simulink model "PV_MEV"  (R2025a)
settings: Solver=VariableStepAuto  StartTime=0.0  StopTime=1  RelTol=1e-3
InitFcn:
  | init_paras
undefined symbols (not defined in the file): C_PFC, D1, Delta, DiscIntNeverNeededParam, ENABLE_HIL, estimation_src, Fnom, Fr_I, Ki_V, Kp_I, Kp_V, Kr_I, L_PFC, Limit_V, mm_10cycle_points, mm_fund_freq, mm_points_per_cycle, RL_PFC, Ro, Ts_Control, Ts_Power, use_d_predict, use_harmonic, use_p_predict, Vnom_ac
libraries: spsSeriesRLCBranchLib x17, spsMeanLib x16, spsCurrentMeasurementLib x9, spsFourierLib x8, spsTHDLib x8, spsVoltageMeasurementLib x8, spsDiodeLib x7, MyLibrary x6, instrumentlib x6, pycoexlib x6, simulink x6, spsPWMGeneratorDCDCLib x4
(part 3 of 6)

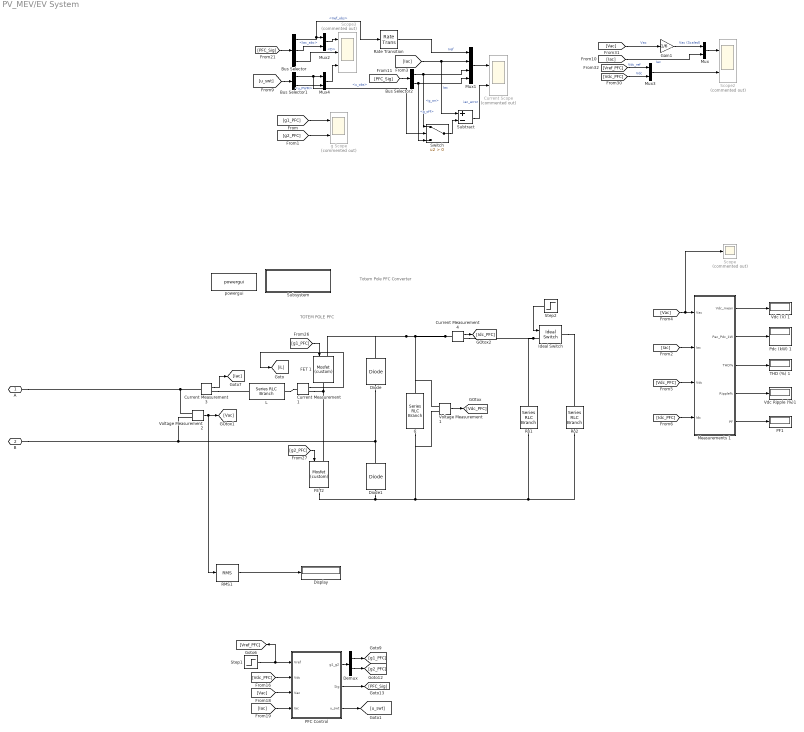
== system PV_MEV/EV System ==
  note: TOTEM POLE PFC
  note: Totem Pole PFC Converter
  Bus Selector : BusSelector  OutputSignals=Iref_obs,Iac_abc,D
  Bus Selector1 : BusSelector  OutputSignals=u_obs,u_PWM
  Bus Selector2 : BusSelector  OutputSignals=g_on,g_off
  C : spsSeriesRLCBranchLib/Series RLC Branch  LConnTagsString=__new0  RConnTagsString=__new0  BranchType=C  Resistance=1  Inductance=1e-3  SetiL0=off  InitialCurrent=0  Capacitance=C_PFC  Setx0=on  InitialVoltage=375  Measurements=None
  Current Measurement1 : spsCurrentMeasurementLib/Current Measurement  PhasorSimulation=off  OutputType=Complex  PSBequivalent=0
  Current Measurement3 : spsCurrentMeasurementLib/Current Measurement  PhasorSimulation=off  OutputType=Complex  PSBequivalent=0
  Current Measurement4 : spsCurrentMeasurementLib/Current Measurement  PhasorSimulation=off  OutputType=Complex  PSBequivalent=0
  Current Scope : Scope  Commented=on  NumInputPorts=2
      settings: ActiveDisplayYMinimum=-76.3871  ActiveDisplayYMaximum=79.5142  DataLoggingSaveFormat=Array
  Demux : Demux  Outputs=2
  Diode : spsDiodeLib/Diode  Ron=Ron_Diode  Lon=0  Vf=Vf  IC=0  UseSnubber=0  Rs=1e6  Cs=inf  Measurements=off
  Diode1 : spsDiodeLib/Diode  Ron=Ron_Diode  Lon=0  Vf=Vf  IC=0  UseSnubber=0  Rs=1e6  Cs=inf  Measurements=off
  Display : Display
  FET 1 : MyLibrary/Mosfet (custom)  Ron=Ron_FET  Lon=0  Rd=Ron_Diode  Vfd=Vf  IC=0  Rs=1e6  Cs=inf  Measurements=off
  FET2 : MyLibrary/Mosfet (custom)  Ron=Ron_FET  Lon=0  Rd=Ron_Diode  Vfd=Vf  IC=0  Rs=1e6  Cs=inf  Measurements=off
  Gain1 : Gain  Gain=1/6
  Ideal Switch : spsIdealSwitchLib/Ideal Switch  Ron=0.001  Lon=0  IC=0  Rs=1e5  Cs=inf  Measurements=off
  L : spsSeriesRLCBranchLib/Series RLC Branch  LConnTagsString=__new0  RConnTagsString=__new0  BranchType=RL  Resistance=RL_PFC  Inductance=L_PFC  SetiL0=off  InitialCurrent=0  Capacitance=1e-6  Setx0=off  InitialVoltage=0  Measurements=None
  Measurements 1 : Subsystem
  Mux{,2..4} (4 alike) : Mux  Inputs=2
  Mux1 : Mux
  PF1 : Display
      settings: Format=bank  Decimation=100
  PFC Control : Subsystem
  Pdc (kW) 1 : Display
      settings: Format=bank  Decimation=100
  RMS1 : spsRMSLib/RMS  TrueRMS=on  Freq=60  RMSInit=0  Ts=5E-08
  Rate Transition : RateTransition
  Ro1 : spsSeriesRLCBranchLib/Series RLC Branch  LConnTagsString=__new0  RConnTagsString=__new0  BranchType=R  Resistance=Ro*2  Inductance=200e-6  SetiL0=off  InitialCurrent=0  Capacitance=400e-6  Setx0=off  InitialVoltage=0  Measurements=None
  Ro2 : spsSeriesRLCBranchLib/Series RLC Branch  LConnTagsString=__new0  RConnTagsString=__new0  BranchType=R  Resistance=Ro*2  Inductance=200e-6  SetiL0=off  InitialCurrent=0  Capacitance=400e-6  Setx0=off  InitialVoltage=0  Measurements=None
  Scope : Scope  Commented=on
      settings: ActiveDisplayYMinimum=193.54878166788092  ActiveDisplayYMaximum=209.93761298828721  DataLoggingVariableName=ScopeData2  DataLoggingSaveFormat=Array
  Scope2 : Scope  Commented=on  NumInputPorts=2
      settings: ActiveDisplayYMinimum=-127.2219  ActiveDisplayYMaximum=127.2109  DataLoggingVariableName=ScopeData3  DataLoggingSaveFormat=Array
  Scope3 : Scope  Commented=on  NumInputPorts=3
      settings: ActiveDisplayYMinimum=-13.4274  ActiveDisplayYMaximum=110.8467  DataLoggingVariableName=ScopeData4  DataLoggingSaveFormat=Array
  Step1 : Step  Time=0.2  Before=350  After=400  SampleTime=Ts_Power
  Step2 : Step  Time=0.4  SampleTime=Ts_Power
  Subsystem : Subsystem
      settings: OpenFcn=edit('Totem_Pole_PFC_v1_data');
      mask Display: disp('Double-click to open\n parameters file');
  Subtract : Sum  Inputs=+-
  Switch : Switch  Criteria=u2 > Threshold  SaturateOnIntegerOverflow=off  InputSameDT=off
  THD (%) 1 : Display
      settings: Format=bank  Decimation=100
  Vdc (V) 1 : Display
      settings: Format=bank  Decimation=100
  Vdc Ripple (%)1 : Display
      settings: Format=bank  Decimation=100
  Voltage Measurement1 : spsVoltageMeasurementLib/Voltage Measurement  PhasorSimulation=off  OutputType=Complex  PSBequivalent=0
  Voltage Measurement2 : spsVoltageMeasurementLib/Voltage Measurement  PhasorSimulation=off  OutputType=Complex  PSBequivalent=0
  g Scope : Scope  Commented=on  NumInputPorts=2
      settings: ActiveDisplayYMinimum=-0.125  ActiveDisplayYMaximum=1.125  DataLoggingVariableName=ScopeData5  DataLoggingSaveFormat=Array
  powergui : spspowerguiLib/powergui  Priority=1  SimulationMode=Discrete  SampleTime=Ts_Power  frequency=60  Iterations=50  frequencyindice=0  Pbase=100e6  ErrMax=1e-4  UnitsV=kV  UnitsW=MW  buscounter=0  FunctionMessages=off  echomessages=off  EnableUseOfTLC=off  CurrentSourceSwitches=off  DisableSnubberDevices=off  DisableRonSwitches=off  DisableVfSwitches=off  DisplayEquations=off  AutomaticDiscreteSolvers=off  SolverType=Tustin/Backward Euler (TBE)  Interpol=off  ExternalGateDelay=off  methode=off  Ts=100  x0status=blocks  SPID=on  SwTol=0  HookPort=off  NonlinearTolerance=1e-4  nMaxIteration=100  ContinueOnMaxIteration=off  RestoreLinks=warning  ResistiveCurrentMeasurement=off  Frange=[0:2:500]  Ylog=off  Xlog=on  ShowGrid=off  save=off  variable=ZData  structure=0  ZoomFFT=off  StartTime=0.0  cycles=1  DisplayStyle=1  fundamental=60  FreqAxis=off  MaxFrequency=1000  frequencyindicesteady=1  RmsSteady=1  display=off
  A : PMIOPort  Side=Left
  B : PMIOPort  Port=2  Side=Left
  wires:
  Bus Selector1/1 -> Mux4/1, Switch/2  "<u_obs>"
  Bus Selector/2 -> Mux2/2  "<Iac_abc>"
  Step1/1 -> PFC Control/1(Vref), [Vref_PFC]
  [g2_PFC] -> FET2/1
  [Iac] -> Measurements 1/2(Iac)
  Bus Selector/3 -> Scope3/2  "<D>"
  [g1_PFC] -> g Scope/1
  Measurements 1/3(THD%) -> THD (%) 1/1
  Voltage Measurement2/1 -> RMS1/1, [Vac]
  Mux3/1 -> Scope2/2
  Measurements 1/4(Ripple%) -> Vdc Ripple (%)1/1
  PFC Control/1(g1_g2) -> Demux/1
  PFC Control/3(u_swt) -> [u_swt]
  Bus Selector2/2 -> Mux1/4, Switch/3  "<g_off>"
  Mux2/1 -> Scope3/1
  Measurements 1/2(Pac_Pdc_kW) -> Pdc (kW) 1/1
  Step2/1 -> Ideal Switch/1
  [Idc_PFC] -> Measurements 1/4(Idc)
  [Iac] -> Subtract/1, Mux1/2  "Iac"
  Gain1/1 -> Mux/1  "Vac (Scaled)"
  [u_swt] -> Bus Selector1/1
  Bus Selector/1 -> Rate Transition/1, Mux2/1  "<Iref_obs>"
  Measurements 1/1(Vdc_mean) -> Vdc (V) 1/1
  [g2_PFC] -> g Scope/2
  [PFC_Sig] -> Bus Selector2/1
  [Vac] -> Scope/1, Measurements 1/1(Vac)
  [Vac] -> Gain1/1  "Vac"
  PFC Control/2(Sig) -> [PFC_Sig]
  [PFC_Sig] -> Bus Selector/1
  [Vdc_PFC] -> PFC Control/2(Vdc)
  Voltage Measurement1/1 -> [Vdc_PFC]
  [g1_PFC] -> FET 1/1
  [Vac] -> PFC Control/3(Vac)
  [Vdc_PFC] -> Measurements 1/3(Vdc)
  Mux/1 -> Scope2/1
  Bus Selector1/2 -> Mux4/2  "<u_PWM>"
  RMS1/1 -> Display/1
  Current Measurement3/1 -> [Iac]
  [Iac] -> Mux/2  "Iac"
  Bus Selector2/1 -> Switch/1, Mux1/3  "<g_on>"
  Switch/1 -> Subtract/2
  Current Measurement1/1 -> [iL]
  [Iac] -> PFC Control/4(Iac)
  Mux4/1 -> Scope3/3
  [Vdc_PFC] -> Mux3/2  "Vdc"
  Demux/1 -> [g1_PFC]
  Demux/2 -> [g2_PFC]
  Rate Transition/1 -> Mux1/1  "Iref"
  Measurements 1/5(PF) -> PF1/1
  Mux1/1 -> Current Scope/1
  [Vref_PFC] -> Mux3/1  "Vdc_ref"
  Subtract/1 -> Current Scope/2  "iac_error"
  Current Measurement4/1 -> [Idc_PFC]
  connections:
  Ideal Switch/LConn1 -- Ro1/LConn1 -- Current Measurement4/RConn1
  Current Measurement1/RConn1 -- FET2/LConn1 -- FET 1/RConn1
  Ro2/RConn1 -- Ro1/RConn1 -- C/RConn1 -- Voltage Measurement1/LConn2 -- FET2/RConn1 -- Diode1/LConn1
  Voltage Measurement2/LConn2 -- B/RConn1 -- Diode/LConn1 -- Diode1/RConn1
  Current Measurement4/LConn1 -- Voltage Measurement1/LConn1 -- C/LConn1 -- Diode/RConn1 -- FET 1/LConn1
  Voltage Measurement2/LConn1 -- A/RConn1 -- Current Measurement3/LConn1
  Current Measurement3/RConn1 -- L/LConn1
  L/RConn1 -- Current Measurement1/LConn1
  Ideal Switch/RConn1 -- Ro2/LConn1

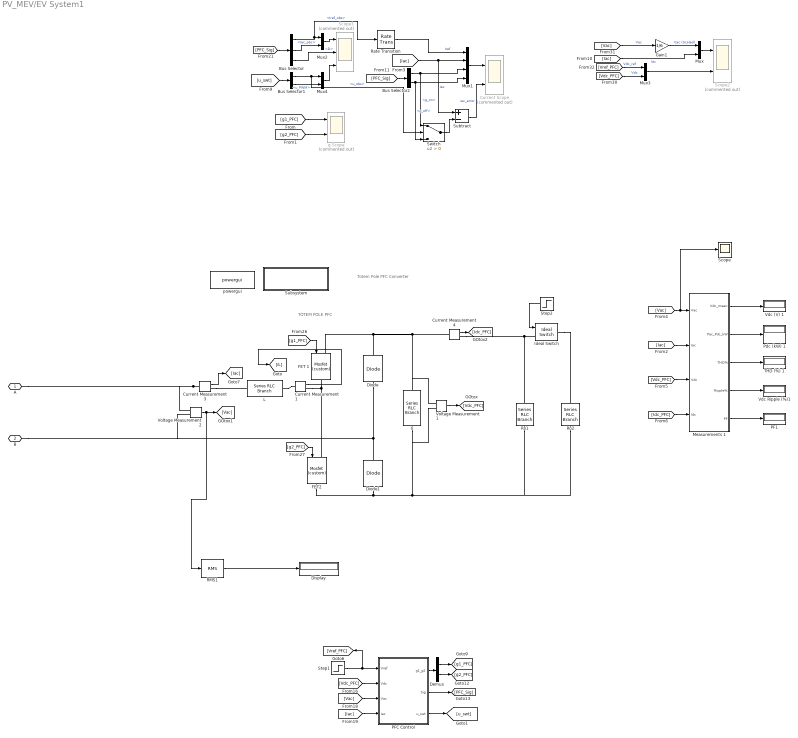
== system PV_MEV/EV System1 ==
  note: Totem Pole PFC Converter
  note: TOTEM POLE PFC
  Bus Selector : BusSelector  OutputSignals=Iref_obs,Iac_abc,D
  Bus Selector1 : BusSelector  OutputSignals=u_obs,u_PWM
  Bus Selector2 : BusSelector  OutputSignals=g_on,g_off
  C : spsSeriesRLCBranchLib/Series RLC Branch  LConnTagsString=__new0  RConnTagsString=__new0  BranchType=C  Resistance=1  Inductance=1e-3  SetiL0=off  InitialCurrent=0  Capacitance=C_PFC  Setx0=on  InitialVoltage=375  Measurements=None
  Current Measurement1 : spsCurrentMeasurementLib/Current Measurement  PhasorSimulation=off  OutputType=Complex  PSBequivalent=0
  Current Measurement3 : spsCurrentMeasurementLib/Current Measurement  PhasorSimulation=off  OutputType=Complex  PSBequivalent=0
  Current Measurement4 : spsCurrentMeasurementLib/Current Measurement  PhasorSimulation=off  OutputType=Complex  PSBequivalent=0
  Current Scope : Scope  Commented=on  NumInputPorts=2
      settings: ActiveDisplayYMinimum=-76.3871  ActiveDisplayYMaximum=79.5142  DataLoggingSaveFormat=Array
  Demux : Demux  Outputs=2
  Diode : spsDiodeLib/Diode  Ron=Ron_Diode  Lon=0  Vf=Vf  IC=0  UseSnubber=0  Rs=1e6  Cs=inf  Measurements=off
  Diode1 : spsDiodeLib/Diode  Ron=Ron_Diode  Lon=0  Vf=Vf  IC=0  UseSnubber=0  Rs=1e6  Cs=inf  Measurements=off
  Display : Display
  FET 1 : MyLibrary/Mosfet (custom)  Ron=Ron_FET  Lon=0  Rd=Ron_Diode  Vfd=Vf  IC=0  Rs=1e6  Cs=inf  Measurements=off
  FET2 : MyLibrary/Mosfet (custom)  Ron=Ron_FET  Lon=0  Rd=Ron_Diode  Vfd=Vf  IC=0  Rs=1e6  Cs=inf  Measurements=off
  Gain1 : Gain  Gain=1/6
  Ideal Switch : spsIdealSwitchLib/Ideal Switch  Ron=0.001  Lon=0  IC=0  Rs=1e5  Cs=inf  Measurements=off
  L : spsSeriesRLCBranchLib/Series RLC Branch  LConnTagsString=__new0  RConnTagsString=__new0  BranchType=RL  Resistance=RL_PFC  Inductance=L_PFC  SetiL0=off  InitialCurrent=0  Capacitance=1e-6  Setx0=off  InitialVoltage=0  Measurements=None
  Measurements 1 : Subsystem
  Mux{,2..4} (4 alike) : Mux  Inputs=2
  Mux1 : Mux
  PF1 : Display
      settings: Format=bank  Decimation=100
  PFC Control : Subsystem
  Pdc (kW) 1 : Display
      settings: Format=bank  Decimation=100
  RMS1 : spsRMSLib/RMS  TrueRMS=on  Freq=60  RMSInit=0  Ts=5E-08
  Rate Transition : RateTransition
  Ro1 : spsSeriesRLCBranchLib/Series RLC Branch  LConnTagsString=__new0  RConnTagsString=__new0  BranchType=R  Resistance=Ro*2  Inductance=200e-6  SetiL0=off  InitialCurrent=0  Capacitance=400e-6  Setx0=off  InitialVoltage=0  Measurements=None
  Ro2 : spsSeriesRLCBranchLib/Series RLC Branch  LConnTagsString=__new0  RConnTagsString=__new0  BranchType=R  Resistance=Ro*2  Inductance=200e-6  SetiL0=off  InitialCurrent=0  Capacitance=400e-6  Setx0=off  InitialVoltage=0  Measurements=None
  Scope : Scope
      settings: DataLoggingVariableName=ScopeData2  DataLoggingSaveFormat=Array
  Scope2 : Scope  Commented=on  NumInputPorts=2
      settings: ActiveDisplayYMinimum=-127.2219  ActiveDisplayYMaximum=127.2109  DataLoggingVariableName=ScopeData3  DataLoggingSaveFormat=Array
  Scope3 : Scope  Commented=on  NumInputPorts=3
      settings: ActiveDisplayYMinimum=-13.4274  ActiveDisplayYMaximum=110.8467  DataLoggingVariableName=ScopeData4  DataLoggingSaveFormat=Array
  Step1 : Step  Time=0.2  Before=350  After=400  SampleTime=Ts_Power
  Step2 : Step  Time=0.4  SampleTime=Ts_Power
  Subsystem : Subsystem
      settings: OpenFcn=edit('Totem_Pole_PFC_v1_data');
      mask Display: disp('Double-click to open\n parameters file');
  Subtract : Sum  Inputs=+-
  Switch : Switch  Criteria=u2 > Threshold  SaturateOnIntegerOverflow=off  InputSameDT=off
  THD (%) 1 : Display
      settings: Format=bank  Decimation=100
  Vdc (V) 1 : Display
      settings: Format=bank  Decimation=100
  Vdc Ripple (%)1 : Display
      settings: Format=bank  Decimation=100
  Voltage Measurement1 : spsVoltageMeasurementLib/Voltage Measurement  PhasorSimulation=off  OutputType=Complex  PSBequivalent=0
  Voltage Measurement2 : spsVoltageMeasurementLib/Voltage Measurement  PhasorSimulation=off  OutputType=Complex  PSBequivalent=0
  g Scope : Scope  Commented=on  NumInputPorts=2
      settings: ActiveDisplayYMinimum=-0.125  ActiveDisplayYMaximum=1.125  DataLoggingVariableName=ScopeData5  DataLoggingSaveFormat=Array
  powergui : spspowerguiLib/powergui  Priority=1  SimulationMode=Discrete  SampleTime=Ts_Power  frequency=60  Iterations=50  frequencyindice=0  Pbase=100e6  ErrMax=1e-4  UnitsV=kV  UnitsW=MW  buscounter=0  FunctionMessages=off  echomessages=off  EnableUseOfTLC=off  CurrentSourceSwitches=off  DisableSnubberDevices=off  DisableRonSwitches=off  DisableVfSwitches=off  DisplayEquations=off  AutomaticDiscreteSolvers=off  SolverType=Tustin/Backward Euler (TBE)  Interpol=off  ExternalGateDelay=off  methode=off  Ts=100  x0status=blocks  SPID=on  SwTol=0  HookPort=off  NonlinearTolerance=1e-4  nMaxIteration=100  ContinueOnMaxIteration=off  RestoreLinks=warning  ResistiveCurrentMeasurement=off  Frange=[0:2:500]  Ylog=off  Xlog=on  ShowGrid=off  save=off  variable=ZData  structure=0  ZoomFFT=off  StartTime=0.0  cycles=1  DisplayStyle=1  fundamental=60  FreqAxis=off  MaxFrequency=1000  frequencyindicesteady=1  RmsSteady=1  display=off
  A : PMIOPort  Side=Left
  B : PMIOPort  Port=2  Side=Left
  wires:
  Current Measurement4/1 -> [Idc_PFC]
  Subtract/1 -> Current Scope/2  "iac_error"
  [Vref_PFC] -> Mux3/1  "Vdc_ref"
  Mux1/1 -> Current Scope/1
  Measurements 1/5(PF) -> PF1/1
  Rate Transition/1 -> Mux1/1  "Iref"
  Demux/2 -> [g2_PFC]
  Demux/1 -> [g1_PFC]
  [Vdc_PFC] -> Mux3/2  "Vdc"
  Mux4/1 -> Scope3/3
  [Iac] -> PFC Control/4(Iac)
  Current Measurement1/1 -> [iL]
  Switch/1 -> Subtract/2
  Bus Selector2/1 -> Mux1/3, Switch/1  "<g_on>"
  [Iac] -> Mux/2  "Iac"
  Current Measurement3/1 -> [Iac]
  RMS1/1 -> Display/1
  Bus Selector1/2 -> Mux4/2  "<u_PWM>"
  Mux/1 -> Scope2/1
  [Vdc_PFC] -> Measurements 1/3(Vdc)
  [Vac] -> PFC Control/3(Vac)
  [g1_PFC] -> FET 1/1
  Voltage Measurement1/1 -> [Vdc_PFC]
  [Vdc_PFC] -> PFC Control/2(Vdc)
  [PFC_Sig] -> Bus Selector/1
  PFC Control/2(Sig) -> [PFC_Sig]
  [Vac] -> Gain1/1  "Vac"
  [Vac] -> Measurements 1/1(Vac), Scope/1
  [PFC_Sig] -> Bus Selector2/1
  [g2_PFC] -> g Scope/2
  Measurements 1/1(Vdc_mean) -> Vdc (V) 1/1
  Bus Selector/1 -> Mux2/1, Rate Transition/1  "<Iref_obs>"
  [u_swt] -> Bus Selector1/1
  Gain1/1 -> Mux/1  "Vac (Scaled)"
  [Iac] -> Mux1/2, Subtract/1  "Iac"
  [Idc_PFC] -> Measurements 1/4(Idc)
  Step2/1 -> Ideal Switch/1
  Measurements 1/2(Pac_Pdc_kW) -> Pdc (kW) 1/1
  Mux2/1 -> Scope3/1
  Bus Selector2/2 -> Switch/3, Mux1/4  "<g_off>"
  PFC Control/3(u_swt) -> [u_swt]
  PFC Control/1(g1_g2) -> Demux/1
  Measurements 1/4(Ripple%) -> Vdc Ripple (%)1/1
  Mux3/1 -> Scope2/2
  Voltage Measurement2/1 -> [Vac], RMS1/1
  Measurements 1/3(THD%) -> THD (%) 1/1
  [g1_PFC] -> g Scope/1
  Bus Selector/3 -> Scope3/2  "<D>"
  [Iac] -> Measurements 1/2(Iac)
  [g2_PFC] -> FET2/1
  Step1/1 -> [Vref_PFC], PFC Control/1(Vref)
  Bus Selector/2 -> Mux2/2  "<Iac_abc>"
  Bus Selector1/1 -> Switch/2, Mux4/1  "<u_obs>"
  connections:
  Ideal Switch/RConn1 -- Ro2/LConn1
  L/RConn1 -- Current Measurement1/LConn1
  Current Measurement3/RConn1 -- L/LConn1
  Current Measurement3/LConn1 -- A/RConn1 -- Voltage Measurement2/LConn1
  FET 1/LConn1 -- Diode/RConn1 -- C/LConn1 -- Voltage Measurement1/LConn1 -- Current Measurement4/LConn1
  Diode1/RConn1 -- Diode/LConn1 -- B/RConn1 -- Voltage Measurement2/LConn2
  Diode1/LConn1 -- FET2/RConn1 -- Voltage Measurement1/LConn2 -- C/RConn1 -- Ro1/RConn1 -- Ro2/RConn1
  FET 1/RConn1 -- FET2/LConn1 -- Current Measurement1/RConn1
  Current Measurement4/RConn1 -- Ro1/LConn1 -- Ideal Switch/LConn1

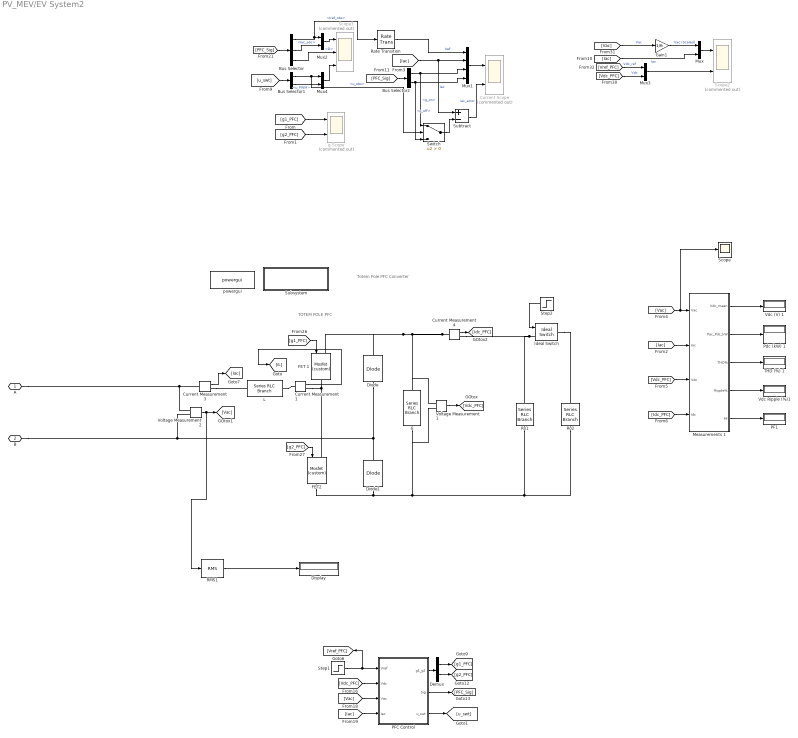
== system PV_MEV/EV System2 ==
  note: TOTEM POLE PFC
  note: Totem Pole PFC Converter
  Bus Selector : BusSelector  OutputSignals=Iref_obs,Iac_abc,D
  Bus Selector1 : BusSelector  OutputSignals=u_obs,u_PWM
  Bus Selector2 : BusSelector  OutputSignals=g_on,g_off
  C : spsSeriesRLCBranchLib/Series RLC Branch  LConnTagsString=__new0  RConnTagsString=__new0  BranchType=C  Resistance=1  Inductance=1e-3  SetiL0=off  InitialCurrent=0  Capacitance=C_PFC  Setx0=on  InitialVoltage=375  Measurements=None
  Current Measurement1 : spsCurrentMeasurementLib/Current Measurement  PhasorSimulation=off  OutputType=Complex  PSBequivalent=0
  Current Measurement3 : spsCurrentMeasurementLib/Current Measurement  PhasorSimulation=off  OutputType=Complex  PSBequivalent=0
  Current Measurement4 : spsCurrentMeasurementLib/Current Measurement  PhasorSimulation=off  OutputType=Complex  PSBequivalent=0
  Current Scope : Scope  Commented=on  NumInputPorts=2
      settings: ActiveDisplayYMinimum=-76.3871  ActiveDisplayYMaximum=79.5142  DataLoggingSaveFormat=Array
  Demux : Demux  Outputs=2
  Diode : spsDiodeLib/Diode  Ron=Ron_Diode  Lon=0  Vf=Vf  IC=0  UseSnubber=0  Rs=1e6  Cs=inf  Measurements=off
  Diode1 : spsDiodeLib/Diode  Ron=Ron_Diode  Lon=0  Vf=Vf  IC=0  UseSnubber=0  Rs=1e6  Cs=inf  Measurements=off
  Display : Display
  FET 1 : MyLibrary/Mosfet (custom)  Ron=Ron_FET  Lon=0  Rd=Ron_Diode  Vfd=Vf  IC=0  Rs=1e6  Cs=inf  Measurements=off
  FET2 : MyLibrary/Mosfet (custom)  Ron=Ron_FET  Lon=0  Rd=Ron_Diode  Vfd=Vf  IC=0  Rs=1e6  Cs=inf  Measurements=off
  Gain1 : Gain  Gain=1/6
  Ideal Switch : spsIdealSwitchLib/Ideal Switch  Ron=0.001  Lon=0  IC=0  Rs=1e5  Cs=inf  Measurements=off
  L : spsSeriesRLCBranchLib/Series RLC Branch  LConnTagsString=__new0  RConnTagsString=__new0  BranchType=RL  Resistance=RL_PFC  Inductance=L_PFC  SetiL0=off  InitialCurrent=0  Capacitance=1e-6  Setx0=off  InitialVoltage=0  Measurements=None
  Measurements 1 : Subsystem
  Mux{,2..4} (4 alike) : Mux  Inputs=2
  Mux1 : Mux
  PF1 : Display
      settings: Format=bank  Decimation=100
  PFC Control : Subsystem
  Pdc (kW) 1 : Display
      settings: Format=bank  Decimation=100
  RMS1 : spsRMSLib/RMS  TrueRMS=on  Freq=60  RMSInit=0  Ts=5E-08
  Rate Transition : RateTransition
  Ro1 : spsSeriesRLCBranchLib/Series RLC Branch  LConnTagsString=__new0  RConnTagsString=__new0  BranchType=R  Resistance=Ro*2  Inductance=200e-6  SetiL0=off  InitialCurrent=0  Capacitance=400e-6  Setx0=off  InitialVoltage=0  Measurements=None
  Ro2 : spsSeriesRLCBranchLib/Series RLC Branch  LConnTagsString=__new0  RConnTagsString=__new0  BranchType=R  Resistance=Ro*2  Inductance=200e-6  SetiL0=off  InitialCurrent=0  Capacitance=400e-6  Setx0=off  InitialVoltage=0  Measurements=None
  Scope : Scope
      settings: DataLoggingVariableName=ScopeData2  DataLoggingSaveFormat=Array
  Scope2 : Scope  Commented=on  NumInputPorts=2
      settings: ActiveDisplayYMinimum=-127.2219  ActiveDisplayYMaximum=127.2109  DataLoggingVariableName=ScopeData3  DataLoggingSaveFormat=Array
  Scope3 : Scope  Commented=on  NumInputPorts=3
      settings: ActiveDisplayYMinimum=-13.4274  ActiveDisplayYMaximum=110.8467  DataLoggingVariableName=ScopeData4  DataLoggingSaveFormat=Array
  Step1 : Step  Time=0.2  Before=350  After=400  SampleTime=Ts_Power
  Step2 : Step  Time=0.4  SampleTime=Ts_Power
  Subsystem : Subsystem
      settings: OpenFcn=edit('Totem_Pole_PFC_v1_data');
      mask Display: disp('Double-click to open\n parameters file');
  Subtract : Sum  Inputs=+-
  Switch : Switch  Criteria=u2 > Threshold  SaturateOnIntegerOverflow=off  InputSameDT=off
  THD (%) 1 : Display
      settings: Format=bank  Decimation=100
  Vdc (V) 1 : Display
      settings: Format=bank  Decimation=100
  Vdc Ripple (%)1 : Display
      settings: Format=bank  Decimation=100
  Voltage Measurement1 : spsVoltageMeasurementLib/Voltage Measurement  PhasorSimulation=off  OutputType=Complex  PSBequivalent=0
  Voltage Measurement2 : spsVoltageMeasurementLib/Voltage Measurement  PhasorSimulation=off  OutputType=Complex  PSBequivalent=0
  g Scope : Scope  Commented=on  NumInputPorts=2
      settings: ActiveDisplayYMinimum=-0.125  ActiveDisplayYMaximum=1.125  DataLoggingVariableName=ScopeData5  DataLoggingSaveFormat=Array
  powergui : spspowerguiLib/powergui  Priority=1  SimulationMode=Discrete  SampleTime=Ts_Power  frequency=60  Iterations=50  frequencyindice=0  Pbase=100e6  ErrMax=1e-4  UnitsV=kV  UnitsW=MW  buscounter=0  FunctionMessages=off  echomessages=off  EnableUseOfTLC=off  CurrentSourceSwitches=off  DisableSnubberDevices=off  DisableRonSwitches=off  DisableVfSwitches=off  DisplayEquations=off  AutomaticDiscreteSolvers=off  SolverType=Tustin/Backward Euler (TBE)  Interpol=off  ExternalGateDelay=off  methode=off  Ts=100  x0status=blocks  SPID=on  SwTol=0  HookPort=off  NonlinearTolerance=1e-4  nMaxIteration=100  ContinueOnMaxIteration=off  RestoreLinks=warning  ResistiveCurrentMeasurement=off  Frange=[0:2:500]  Ylog=off  Xlog=on  ShowGrid=off  save=off  variable=ZData  structure=0  ZoomFFT=off  StartTime=0.0  cycles=1  DisplayStyle=1  fundamental=60  FreqAxis=off  MaxFrequency=1000  frequencyindicesteady=1  RmsSteady=1  display=off
  A : PMIOPort  Side=Left
  B : PMIOPort  Port=2  Side=Left
  wires:
  Bus Selector1/1 -> Mux4/1, Switch/2  "<u_obs>"
  Bus Selector/2 -> Mux2/2  "<Iac_abc>"
  Step1/1 -> PFC Control/1(Vref), [Vref_PFC]
  [g2_PFC] -> FET2/1
  [Iac] -> Measurements 1/2(Iac)
  Bus Selector/3 -> Scope3/2  "<D>"
  [g1_PFC] -> g Scope/1
  Measurements 1/3(THD%) -> THD (%) 1/1
  Voltage Measurement2/1 -> RMS1/1, [Vac]
  Mux3/1 -> Scope2/2
  Measurements 1/4(Ripple%) -> Vdc Ripple (%)1/1
  PFC Control/1(g1_g2) -> Demux/1
  PFC Control/3(u_swt) -> [u_swt]
  Bus Selector2/2 -> Mux1/4, Switch/3  "<g_off>"
  Mux2/1 -> Scope3/1
  Measurements 1/2(Pac_Pdc_kW) -> Pdc (kW) 1/1
  Step2/1 -> Ideal Switch/1
  [Idc_PFC] -> Measurements 1/4(Idc)
  [Iac] -> Subtract/1, Mux1/2  "Iac"
  Gain1/1 -> Mux/1  "Vac (Scaled)"
  [u_swt] -> Bus Selector1/1
  Bus Selector/1 -> Rate Transition/1, Mux2/1  "<Iref_obs>"
  Measurements 1/1(Vdc_mean) -> Vdc (V) 1/1
  [g2_PFC] -> g Scope/2
  [PFC_Sig] -> Bus Selector2/1
  [Vac] -> Scope/1, Measurements 1/1(Vac)
  [Vac] -> Gain1/1  "Vac"
  PFC Control/2(Sig) -> [PFC_Sig]
  [PFC_Sig] -> Bus Selector/1
  [Vdc_PFC] -> PFC Control/2(Vdc)
  Voltage Measurement1/1 -> [Vdc_PFC]
  [g1_PFC] -> FET 1/1
  [Vac] -> PFC Control/3(Vac)
  [Vdc_PFC] -> Measurements 1/3(Vdc)
  Mux/1 -> Scope2/1
  Bus Selector1/2 -> Mux4/2  "<u_PWM>"
  RMS1/1 -> Display/1
  Current Measurement3/1 -> [Iac]
  [Iac] -> Mux/2  "Iac"
  Bus Selector2/1 -> Switch/1, Mux1/3  "<g_on>"
  Switch/1 -> Subtract/2
  Current Measurement1/1 -> [iL]
  [Iac] -> PFC Control/4(Iac)
  Mux4/1 -> Scope3/3
  [Vdc_PFC] -> Mux3/2  "Vdc"
  Demux/1 -> [g1_PFC]
  Demux/2 -> [g2_PFC]
  Rate Transition/1 -> Mux1/1  "Iref"
  Measurements 1/5(PF) -> PF1/1
  Mux1/1 -> Current Scope/1
  [Vref_PFC] -> Mux3/1  "Vdc_ref"
  Subtract/1 -> Current Scope/2  "iac_error"
  Current Measurement4/1 -> [Idc_PFC]
  connections:
  Ideal Switch/LConn1 -- Ro1/LConn1 -- Current Measurement4/RConn1
  Current Measurement1/RConn1 -- FET2/LConn1 -- FET 1/RConn1
  Ro2/RConn1 -- Ro1/RConn1 -- C/RConn1 -- Voltage Measurement1/LConn2 -- FET2/RConn1 -- Diode1/LConn1
  Voltage Measurement2/LConn2 -- B/RConn1 -- Diode/LConn1 -- Diode1/RConn1
  Current Measurement4/LConn1 -- Voltage Measurement1/LConn1 -- C/LConn1 -- Diode/RConn1 -- FET 1/LConn1
  Voltage Measurement2/LConn1 -- A/RConn1 -- Current Measurement3/LConn1
  Current Measurement3/RConn1 -- L/LConn1
  L/RConn1 -- Current Measurement1/LConn1
  Ideal Switch/RConn1 -- Ro2/LConn1

== system PV_MEV/PV System ==
  note: 100-kW  PV Array
      | 330 * SunPower SPR-305E-WHT-D  (Nser=5 Npar=66)
  10 kvar : spsThreePhaseSeriesRLCLoadLib/Three-Phase Series RLC Load  LConnTagsString=A|B|C  Configuration=Y (grounded)  NominalVoltage=Vnom_ac  Vabc=[1e3 1e3 1e3]  Vabcp=[1e3 1e3 1e3]  NominalFrequency=Fnom  UnbalancedPower=off  ActivePower=10e3/100  InductivePower=0  CapacitivePower=10e3  Pabc=[10e3 9e3 11e3]  QLabc=[100 90 110]  QCabc=[100 90 110]  Pabcp=[10e3 9e3 11e3]  QLabcp=[100 90 110]  QCabcp=[100 90 110]  Measurements=None  LoadType=constant Z
  DC AC Inverter : Subsystem
  DC DC Boost Converter : Subsystem
  L : spsThreePhaseSeriesRLCBranchLib/Three-Phase Series RLC Branch  LConnTagsString=A|B|C  RConnTagsString=A|B|C  BranchType=RL  Resistance=500e-6*377/50/2  Inductance=500e-6/2  Capacitance=inf  Measurements=None
  PV Array : spsPVArrayLib/PV Array  Npar=66  Nser=5  PlotType=array @ 1000 W/m2 & specified temperatures  S_vec="[ 1000  250 ]"  Temp_C_vec="[0 25 50  ]"  ModuleName=SunPower SPR-305E-WHT-D  PlotWhenSelected=off  Pm=305.226  Ncell=96  Voc=64.2  Isc=5.96  Vm=54.7  Im=5.58  beta_Voc_pc=-0.2727  alpha_Isc_pc=0.061745  beta_Voc=-0.17507  alpha_Isc=0.00368  IL=5.9657  I0=6.3076e-12  nI=0.94489  Rsh=393.2054  Rs=0.37428  RobustModel=off  RobustCellTemperature=25  BAL=on  Tc=1e-6  Tfilter=5e-5
  PV Enviroment : Subsystem
  PV Status : Subsystem
  A : PMIOPort  Side=Right
  B : PMIOPort  Port=2  Side=Right
  C : PMIOPort  Port=3  Side=Right
  wires:
  PV Array/1 -> PV Status/1(m_PV)
  PV Enviroment/2(Temp) -> PV Array/2
  PV Enviroment/1(Ir) -> PV Array/1
  connections:
  10 kvar/LConn1 -- A/RConn1 -- L/RConn1
  10 kvar/LConn2 -- B/RConn1 -- L/RConn2
  10 kvar/LConn3 -- C/RConn1 -- L/RConn3
  DC AC Inverter/LConn1 -- DC DC Boost Converter/RConn1
  DC AC Inverter/LConn3 -- DC DC Boost Converter/RConn3
  DC AC Inverter/RConn3 -- L/LConn3
  DC AC Inverter/RConn2 -- L/LConn2
  PV Array/RConn1 -- DC DC Boost Converter/LConn1
  PV Array/RConn2 -- DC DC Boost Converter/LConn2
  DC AC Inverter/LConn2 -- DC DC Boost Converter/RConn2
  DC AC Inverter/RConn1 -- L/LConn1

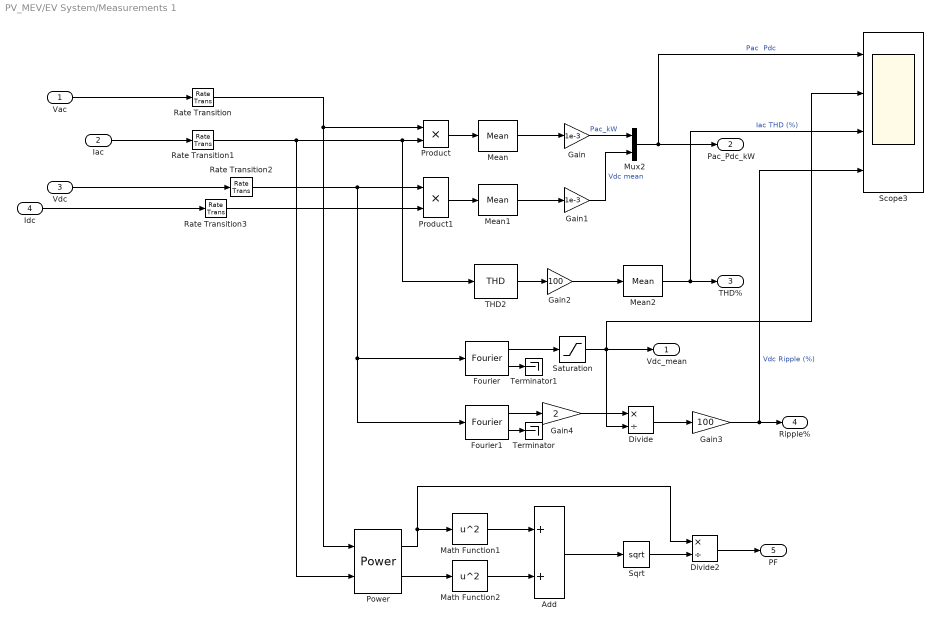
== system PV_MEV/EV System/Measurements 1 ==
  Vac : Inport
  Iac : Inport  Port=2
  Vdc : Inport  Port=3
  Idc : Inport  Port=4
  Add : Sum
  Divide : Product  Inputs=*/
  Divide2 : Product  Inputs=*/
  Fourier : spsFourierLib/Fourier  Freq=Fnom  n=0  InInit=[0, 0]  Ts=Ts_Control
  Fourier1 : spsFourierLib/Fourier  Freq=Fnom  n=2  InInit=[0, 0]  Ts=Ts_Control
  Gain : Gain  Gain=1e-3
  Gain1 : Gain  Gain=1e-3
  Gain2 : Gain  Gain=100
  Gain3 : Gain  Gain=100
  Gain4 : Gain  Gain=2
  Math Function1 : Math  Operator=square
  Math Function2 : Math  Operator=square
  Mean : spsMeanLib/Mean  Freq=Fnom  Vinit=0  Ts=Ts_Control
  Mean1 : spsMeanLib/Mean  Freq=Fnom  Vinit=0  Ts=Ts_Control
  Mean2 : spsMeanLib/Mean  Freq=Fnom  Vinit=0  Ts=Ts_Control
  Mux2 : Mux  Inputs=2
  Power : spsPowerLib/Power  Freq=Fnom  Vinit=[1, 0]  Iinit=[1, 0]  Ts=Ts_Control
  Product : Product
  Product1 : Product
  Rate Transition{,1..3} (4 alike) : RateTransition  OutPortSampleTime=Ts_Control
  Saturation : Saturate  UpperLimit=inf  LowerLimit=eps
  Scope3 : Scope  NumInputPorts=4
      settings: ActiveDisplayYMinimum=0.93708953826649433  ActiveDisplayYMaximum=9.2780325590277677  DataLoggingSaveFormat=Array
  Sqrt : Sqrt
  THD2 : spsTHDLib/THD  Freq=Fnom  Ts=Ts_Control
  Terminator : Terminator
  Terminator1 : Terminator
  Vdc_mean : Outport
  Pac_Pdc_kW : Outport  Port=2
  THD% : Outport  Port=3
  Ripple% : Outport  Port=4
  PF : Outport  Port=5
  wires:
  Gain1/1 -> Mux2/2  "Vdc mean"
  Product1/1 -> Mean1/1
  Mean/1 -> Gain/1
  Product/1 -> Mean/1
  Gain/1 -> Mux2/1  "Pac_kW"
  THD2/1 -> Gain2/1
  Mean1/1 -> Gain1/1
  Iac/1 -> Rate Transition1/1
  Mux2/1 -> Scope3/1, Pac_Pdc_kW/1  "Pac  Pdc"
  Gain2/1 -> Mean2/1
  Mean2/1 -> Scope3/3, THD%/1  "Iac THD (%)"
  Fourier/2 -> Terminator1/1
  Fourier/1 -> Saturation/1
  Saturation/1 -> Scope3/2, Vdc_mean/1, Divide/2
  Divide/1 -> Gain3/1
  Fourier1/1 -> Gain4/1
  Gain4/1 -> Divide/1
  Fourier1/2 -> Terminator/1
  Gain3/1 -> Scope3/4, Ripple%/1  "Vdc Ripple (%)"
  Power/1 -> Math Function1/1, Divide2/1
  Power/2 -> Math Function2/1
  Math Function1/1 -> Add/1
  Math Function2/1 -> Add/2
  Add/1 -> Sqrt/1
  Sqrt/1 -> Divide2/2
  Divide2/1 -> PF/1
  Rate Transition1/1 -> Power/2, THD2/1, Product/2
  Vdc/1 -> Rate Transition2/1
  Idc/1 -> Rate Transition3/1
  Rate Transition/1 -> Power/1, Product/1
  Vac/1 -> Rate Transition/1
  Rate Transition2/1 -> Product1/1, Fourier/1, Fourier1/1
  Rate Transition3/1 -> Product1/2

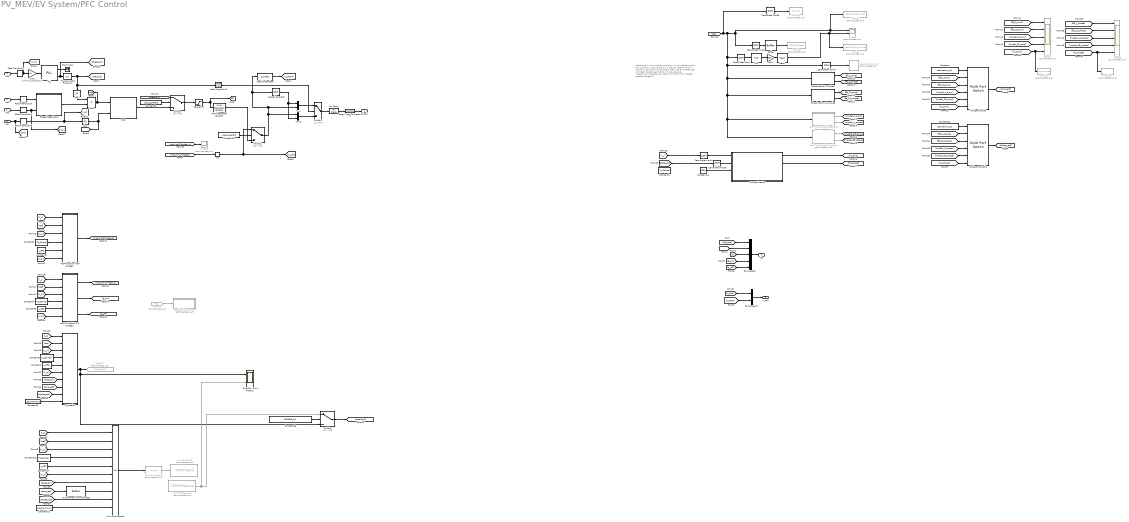
== system PV_MEV/EV System/PFC Control ==
  note: Make sure
      | 1. onnxruntime and onnx in your base python enviroment.
      | 2. reload the onnx file and refresh them in the onnx call block.
      | or comment them like this
      | otherwise will lead matlab crash
      |
      | (bash)
      | conda activate matlab_onnx_py310
      | pip install onnx==1.14.0
      |
      | (matlab console)
      | target = "/home/changhong/anaconda3/envs/matlab_onnx_py310/bin/python";
      | pe = pyenv
      | pyenv("Version", target)
  Vref : Inport
  Vdc : Inport  Port=2
  Vac : Inport  Port=3
  Iac : Inport  Port=4
  AbsI : Abs  SaturateOnIntegerOverflow=off
  AbsV : Abs  SaturateOnIntegerOverflow=off
  Buffer : Buffer  N=80  V=79  OutputFrames=off
  Bus Creator : BusCreator  Inputs=5
  Bus Creator1 : BusCreator  Inputs=2
  Cast To Boolean : DataTypeConversion  OutDataTypeStr=boolean  SaturateOnIntegerOverflow=off  RndMeth=Floor
  Constant : Constant  Value=estimation_src
  Constant{1..2,4,6,13} (5 alike) : Constant  Value=Ts_Control
  Constant10 : Constant  Value=use_p_predict
  Constant11 : Constant  Value=estimation_src
  Constant12 : Constant  Value=4000
  Constant{3,5,7,14} (4 alike) : Constant  Value=L_PFC
  Constant15 : Constant  Value=use_harmonic
  Constant16 : Constant  Value=ENABLE_HIL
  Constant8 : Constant  Value=use_harmonic
  Constant9 : Constant  Value=use_d_predict
  D_predict : MATLAB Function  TreatAsAtomicUnit=on
  Data Type Conversion2 : DataTypeConversion  OutDataTypeStr=double  SaturateOnIntegerOverflow=off  RndMeth=Floor
  Enabled Subsystem : Subsystem  Commented=on  TreatAsAtomicUnit=on
  From49 : From  Commented=on  GotoTag=Iac
  Gain : Gain  Gain=100
  Goto17 : Goto  Commented=on  GotoTag=predict_D
  HIL Harmonic Amplitudes1 : Selector  InputPortWidth=4  IndexOptions=Index vector (dialog)  Indices=[2 3 4]  OutputSizes=1
  HIL Input Frame1 : Mux  Inputs=10
  HIL Input Single1 : DataTypeConversion  Commented=on  OutDataTypeStr=single  SaturateOnIntegerOverflow=off  RndMeth=Floor
  HIL TCP Receive1 : instrumentlib/TCP//IP Receive  Priority=30  Commented=on  Host=134.226.86.100  Port=5011  DataSize=[1, 1]  DataType=single  ASCIIFormatting=%f  Terminator=LF  CustomTerminator=10  ByteOrder=little-endian  EnableBlockingMode=on  Timeout=10  SampleTime=Ts_Control  SimulateUsing=Interpreted execution
  HIL TCP Send1 : instrumentlib/TCP//IP Send  Priority=-30  Commented=on  Host=134.226.86.100  Port=5010  ByteOrder=little-endian  EnableBlockingMode=on  Timeout=10  TransferDelay=off  SimulateUsing=Interpreted execution
  Half Cycle Model Prediction : Subsystem  Commented=on
  Logical Operator : Logic  Operator=NOT  AllPortsSameDT=off  OutDataTypeStr=float('double')
  MCP Function Half bridge1 : MATLAB Function  TreatAsAtomicUnit=on
  Mean : spsMeanLib/Mean  Freq=50  Vinit=0  Ts=1/4000
  Multiport Switch : MultiPortSwitch  Inputs=5  SaturateOnIntegerOverflow=off  InputSameDT=off
  Multiport Switch1 : MultiPortSwitch  Inputs=5  SaturateOnIntegerOverflow=off  InputSameDT=off
  Mux : Mux  Inputs=2
  Mux2 : Mux  Inputs=2
  On Delay : spsOnDelayLib/On Delay  DelayType=On delay  delay=DT_PFC  ic=0  Ts=Ts_Power
  One  Cycle Model Prediction : Subsystem  Commented=on
  Original vs HIL Predict : Scope  NumInputPorts=2
      settings: ActiveDisplayYMinimum=-1.664049084961701E+6  ActiveDisplayYMaximum=2.2609897552756537E+6
  PLL : spsPLLLib/PLL  Fmin=0.9*Fnom  Par_Init=[0, Fnom]  ParK=[180, 3200, 1]  TcD=1e-4  MaxRateChangeFreq=12  FilterCutOffFreq=25  Ts=Ts_Control  AGC=on
  PR2 : Subsystem  mask(Current Regulator (Pr)){Kp=Kp_I, Kr=Kr_I, Fr=Fr_I}
      mask prompts: Kp "Proportional gain"; Kr "Resonant gain"; Fr "Resonant frequency (Hz)"
      mask help: This block implements a currentregulator using a PR controller.
      mask Display: disp('Current Regulator\n PR');
  PWM Generator (DC-DC) : spsPWMGeneratorDCDCLib/PWM Generator (DC-DC)  Fsw=Fsw  Ts=Ts_Power
  Prod1 : Product
  RLS_estimation : MATLAB Function  TreatAsAtomicUnit=on
  RT : RateTransition  OutPortSampleTime=5e-08
  Rate Transition{,3..5} (4 alike) : RateTransition  OutPortSampleTime=Ts_Control
  Rate Transition2 : RateTransition  OutPortSampleTime=Ts_Power
  Saturation : Saturate  UpperLimit=1  LowerLimit=0
  Scope : Scope  Commented=on  NumInputPorts=2
      settings: ActiveDisplayYMinimum=-211.219  ActiveDisplayYMaximum=223.7073  DataLoggingVariableName=ScopeData4  DataLoggingSaveFormat=Array
  Scope1 : Scope  Commented=on  NumInputPorts=5
      settings: ActiveDisplayYMinimum=-19.4864  ActiveDisplayYMaximum=175.3777  DataLoggingVariableName=ScopeData5  DataLoggingSaveFormat=Array
  Scope2 : Scope  Commented=on
      settings: DataLoggingVariableName=ScopeData9  DataLoggingSaveFormat=Array
  Scope3 : Scope  Commented=on  NumInputPorts=5
      settings: ActiveDisplayYMinimum=-3.927  ActiveDisplayYMaximum=3.927  DataLoggingVariableName=ScopeData6  DataLoggingSaveFormat=Array
  Spectrum Analyzer : SpectrumAnalyzer  Commented=on  WindowPosition=[-2559.000000,62.000000,1707.000000,996.000000,]  ScopeFrameLocation=window  SampleRateSource=Property  SampleRate=8000  PlotAsTwoSidedSpectrum=off  WindowInvariantSamplesPerUpdate=on  FrequencySpan=Start and stop frequencies  StartFrequency=0  StopFrequency=2000  YLimits=[-21.57310057,75.63654601]  ColorLimits=[-42.4528 59.157]
  Speed Regulator2 : Subsystem  DialogController=POWERSYS.PowerSysDialog  mask(Voltage Regulator){Kp=Kp_V, Ki=Ki_V, Limit_wreg=Limit_V, Init=0, Ts=Ts_Control}
      mask prompts: Kp "Proportional gain (Kp):"; Ki "Integral gain (Ki):"; Limit_wreg "Output limits"; Init "Output initial value:"; Ts "Sample time:"
      mask help: This block implements a voltage regulator using an ant-windup PI controller.
      mask Display: disp('Voltage\nRegulator');
  Switch : Switch  Criteria=u2 > Threshold  Threshold=0.5  SaturateOnIntegerOverflow=off  InputSameDT=off
  Switch1 : Switch  SaturateOnIntegerOverflow=off  InputSameDT=off
  Switch2 : Switch  Criteria=u2 > Threshold  Threshold=0.5  SaturateOnIntegerOverflow=off  InputSameDT=off
  Switch3 : Switch  Criteria=u2 > Threshold  Threshold=0.5  SaturateOnIntegerOverflow=off  InputSameDT=off
  THD : spsTHDLib/THD  Freq=50  Ts=1/4000
  Terminator : Terminator
  To File : ToFile  Commented=on  Filename=MPCC_IAC.mat  SaveFormat=Timeseries
  To File1 : ToFile  Commented=on  Filename=rls_phase.mat  SaveFormat=Timeseries
  To File2 : ToFile  Commented=on  Filename=rls_amp.mat  SaveFormat=Timeseries
  To File3 : ToFile  Commented=on  Filename=Iac.mat  SaveFormat=Timeseries
  To File4 : ToFile  Commented=on  Filename=results/Iac_ori.mat  SaveFormat=Timeseries
  To File5 : ToFile  Commented=on  Filename=results/THD_ori.mat  SaveFormat=Timeseries
  Trigonometric Function7 : Trigonometry
  UMPC Function Full bridge1 : MATLAB Function  TreatAsAtomicUnit=on
  Zero-Order Hold{,1,3..5} (5 alike) : ZeroOrderHold  SampleTime=1/4000
  Zero-Order Hold2 : ZeroOrderHold  SampleTime=1/8000
  fft estimation 1 cycle2 : Subsystem
  fft estimation 10 cycle2 : Subsystem
  to-pu : Gain  Gain=1/(Vnom_ac*sqrt(2))
  g1_g2 : Outport  PortDimensions=2
  Sig : Outport  Port=2
  u_swt : Outport  Port=3
  wires:
  Mux/1 -> Switch1/1
  Iac/1 -> [Iac], Rate Transition5/1
  Speed Regulator2/1(Out) -> Prod1/2
  Rate Transition2/1 -> Switch1/2
  Data Type Conversion2/1 -> g1_g2/1
  PLL/2 -> [theta_pll], Trigonometric Function7/1
  Saturation/1 -> PWM Generator (DC-DC)/1, [D]
  to-pu/1 -> PLL/1
  Rate Transition/1 -> [V_in], to-pu/1
  Bus Creator1/1 -> u_swt/1
  AbsI/1 -> PR2/2(Iac), [Iac_abs]
  Trigonometric Function7/1 -> AbsV/1, Rate Transition2/1, [Iref_obs]
  [D] -> Bus Creator/3  "D"
  Rate Transition3/1 -> Speed Regulator2/1(Vref)
  Switch1/1 -> On Delay/1
  Rate Transition4/1 -> Speed Regulator2/2(Vmeas), [V_o]
  [u_obs] -> Bus Creator1/1  "u_obs"
  Mux2/1 -> Switch1/3
  Vdc/1 -> Rate Transition4/1
  [mcp_full_bridge_o] -> RT/1
  [Iref_obs] -> Bus Creator/1  "Iref_obs"
  RT/1 -> Switch2/1, [u_obs]
  Cast To Boolean/1 -> [u_PWM]
  PWM Generator (DC-DC)/1 -> Switch2/3
  Vac/1 -> Rate Transition/1
  Prod1/1 -> [Iref], PR2/1(Iref)
  Bus Creator/1 -> Sig/1
  Rate Transition5/1 -> [i_L], AbsI/1
  PLL/1 -> Terminator/1
  AbsV/1 -> Prod1/1
  [Iac_abs] -> Bus Creator/2  "Iac_abc"
  Switch2/1 -> Logical Operator/1, Cast To Boolean/1, Mux/2, Mux2/1
  Vref/1 -> Rate Transition3/1
  On Delay/1 -> Data Type Conversion2/1
  [u_PWM] -> Bus Creator1/2  "u_PWM"
  [Iac] -> Zero-Order Hold3/1, Half Cycle Model Prediction/1(u), One  Cycle Model Prediction/1(u), fft estimation 10 cycle2/1(u), fft estimation 1 cycle2/1(u), Zero-Order Hold2/1, Zero-Order Hold/1, Zero-Order Hold1/1, To File4/1, Scope/1  "Iac"
  Buffer/1 -> To File/1
  Gain/1 -> Mean/1
  Zero-Order Hold/1 -> THD/1
  Mean/1 -> To File5/1, Scope/2
  Zero-Order Hold2/1 -> Spectrum Analyzer/1
  THD/1 -> Gain/1
  Zero-Order Hold1/1 -> Buffer/1
  [i_L] -> MCP Function Half bridge1/1(i_L)
  [Iref] -> MCP Function Half bridge1/2(i_ref)
  [V_in] -> MCP Function Half bridge1/3(V_in)
  Constant2/1 -> MCP Function Half bridge1/4(Ts)
  Constant3/1 -> MCP Function Half bridge1/5(L_in)
  [V_o] -> MCP Function Half bridge1/6(V_o)
  MCP Function Half bridge1/1(y) -> [mcp_half_bridge_o]
  [i_L] -> UMPC Function Full bridge1/1(i_L)
  [Iref] -> UMPC Function Full bridge1/2(i_ref)
  [V_in] -> UMPC Function Full bridge1/3(V_in)
  Constant4/1 -> UMPC Function Full bridge1/4(Ts)
  Constant5/1 -> UMPC Function Full bridge1/5(L_in)
  [V_o] -> UMPC Function Full bridge1/6(V_o)
  UMPC Function Full bridge1/1(y) -> [mcp_full_bridge_o]
  UMPC Function Full bridge1/2(g_on) -> [g_on]
  UMPC Function Full bridge1/3(g_off) -> [g_off]
  [g_on] -> Bus Creator/4  "g_on"
  [g_off] -> Bus Creator/5  "g_off"
  [theta_pll] -> Zero-Order Hold5/1
  [i_L] -> D_predict/1(i_L)
  [Iref] -> D_predict/2(i_ref)
  [V_in] -> D_predict/3(V_in)
  Constant6/1 -> D_predict/4(Ts)
  Constant7/1 -> D_predict/5(L_in)
  [V_o] -> D_predict/6(V_o)
  [amp_est] -> D_predict/8(amp_est)
  [phase_est] -> D_predict/9(phase_est)
  Constant8/1 -> D_predict/10(use_harmonic)
  [theta_pll] -> D_predict/7(theta_pll)
  D_predict/1(D) -> Switch3/3, Original vs HIL Predict/1, Goto17/1
  [mcp_half_bridge_o] -> Scope2/1
  Constant9/1 -> Switch/2
  [predict_D] -> Switch/1
  PR2/1(D) -> Switch/3
  Switch/1 -> Saturation/1
  Constant10/1 -> Switch2/2
  Logical Operator/1 -> Mux2/2, Mux/1
  Constant/1 -> Multiport Switch/1
  fft estimation 1 cycle2/1(amp) -> [fft_1_amp]
  fft estimation 1 cycle2/2(phase) -> [fft_1_phase]
  fft estimation 10 cycle2/1(amp) -> [fft_10_amp]
  fft estimation 10 cycle2/2(phase) -> [fft_10_phase]
  One  Cycle Model Prediction/1(amplitude) -> [model_1_amp]
  One  Cycle Model Prediction/2(phase) -> [model_1_phase]
  Half Cycle Model Prediction/1(amplitude) -> [model_05_amp]  "amp_est"
  Half Cycle Model Prediction/2(phase) -> [model_05_phase]  "hase_est"
  Multiport Switch/1 -> [amp_est]
  RLS_estimation/1(amp_est) -> [rls_amp]
  RLS_estimation/2(phase_est) -> [rls_phase]
  [fft_1_amp] -> Multiport Switch/2
  [fft_10_amp] -> Multiport Switch/3
  [model_1_amp] -> Multiport Switch/4
  [model_05_amp] -> Multiport Switch/5
  [rls_amp] -> Multiport Switch/6
  [rls_phase] -> Multiport Switch1/6
  [model_05_phase] -> Multiport Switch1/5
  [model_1_phase] -> Multiport Switch1/4
  [fft_10_phase] -> Multiport Switch1/3
  [fft_1_phase] -> Multiport Switch1/2
  Multiport Switch1/1 -> [phase_est]
  Constant11/1 -> Multiport Switch1/1
  [fft_1_amp] -> Scope1/1
  [fft_10_amp] -> Scope1/2
  [model_1_amp] -> Scope1/3
  [model_05_amp] -> Scope1/4
  [rls_amp] -> To File2/1, Scope1/5
  [fft_1_phase] -> Scope3/1
  [fft_10_phase] -> Scope3/2
  [model_1_phase] -> Scope3/3
  [model_05_phase] -> Scope3/4
  [rls_phase] -> To File1/1, Scope3/5
  Zero-Order Hold3/1 -> To File3/1
  [i_L] -> Zero-Order Hold4/1
  Constant12/1 -> RLS_estimation/3(Ts)
  Zero-Order Hold4/1 -> RLS_estimation/1(i_L)
  Zero-Order Hold5/1 -> RLS_estimation/2(theta_pll)
  From49/1 -> Enabled Subsystem/1(Iac)  "Iac"
  [amp_est] -> HIL Harmonic Amplitudes1/1
  [i_L] -> HIL Input Frame1/1
  [Iref] -> HIL Input Frame1/2
  [V_in] -> HIL Input Frame1/3
  Constant13/1 -> HIL Input Frame1/4
  Constant14/1 -> HIL Input Frame1/5
  [V_o] -> HIL Input Frame1/6
  [theta_pll] -> HIL Input Frame1/7
  HIL Harmonic Amplitudes1/1 -> HIL Input Frame1/8
  [phase_est] -> HIL Input Frame1/9
  Constant15/1 -> HIL Input Frame1/10
  HIL Input Single1/1 -> HIL TCP Send1/1
  HIL Input Frame1/1 -> HIL Input Single1/1
  HIL TCP Receive1/1 -> Original vs HIL Predict/2, Switch3/1
  Switch3/1 -> [predict_D]
  Constant16/1 -> Switch3/2

== system PV_MEV/EV System/Subsystem ==

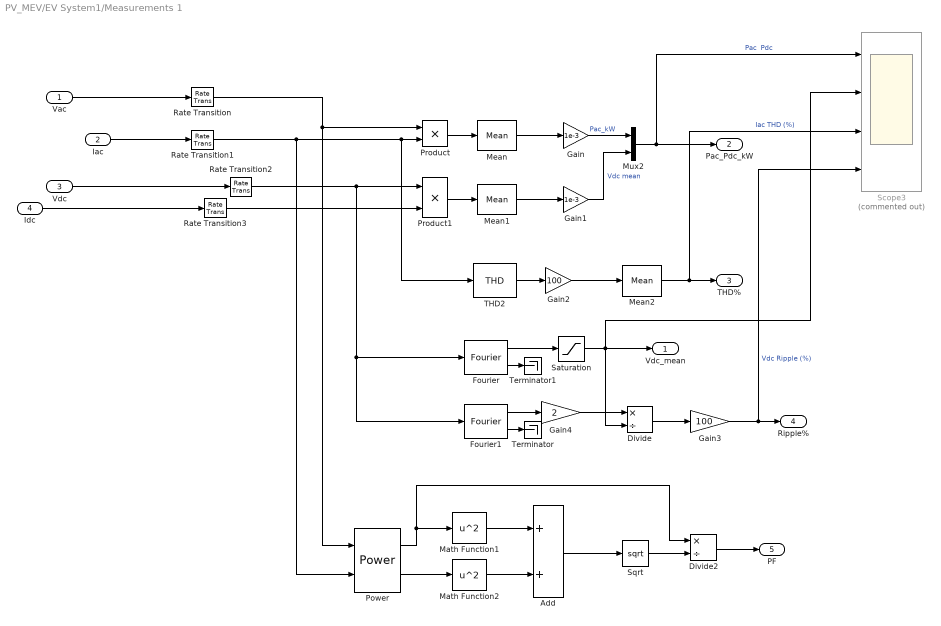
== system PV_MEV/EV System1/Measurements 1 ==
  Vac : Inport
  Iac : Inport  Port=2
  Vdc : Inport  Port=3
  Idc : Inport  Port=4
  Add : Sum
  Divide : Product  Inputs=*/
  Divide2 : Product  Inputs=*/
  Fourier : spsFourierLib/Fourier  Freq=Fnom  n=0  InInit=[0, 0]  Ts=Ts_Control
  Fourier1 : spsFourierLib/Fourier  Freq=Fnom  n=2  InInit=[0, 0]  Ts=Ts_Control
  Gain : Gain  Gain=1e-3
  Gain1 : Gain  Gain=1e-3
  Gain2 : Gain  Gain=100
  Gain3 : Gain  Gain=100
  Gain4 : Gain  Gain=2
  Math Function1 : Math  Operator=square
  Math Function2 : Math  Operator=square
  Mean : spsMeanLib/Mean  Freq=Fnom  Vinit=0  Ts=Ts_Control
  Mean1 : spsMeanLib/Mean  Freq=Fnom  Vinit=0  Ts=Ts_Control
  Mean2 : spsMeanLib/Mean  Freq=Fnom  Vinit=0  Ts=Ts_Control
  Mux2 : Mux  Inputs=2
  Power : spsPowerLib/Power  Freq=Fnom  Vinit=[1, 0]  Iinit=[1, 0]  Ts=Ts_Control
  Product : Product
  Product1 : Product
  Rate Transition{,1..3} (4 alike) : RateTransition  OutPortSampleTime=Ts_Control
  Saturation : Saturate  UpperLimit=inf  LowerLimit=eps
  Scope3 : Scope  Commented=on  NumInputPorts=4
      settings: DataLoggingSaveFormat=Array
  Sqrt : Sqrt
  THD2 : spsTHDLib/THD  Freq=Fnom  Ts=Ts_Control
  Terminator : Terminator
  Terminator1 : Terminator
  Vdc_mean : Outport
  Pac_Pdc_kW : Outport  Port=2
  THD% : Outport  Port=3
  Ripple% : Outport  Port=4
  PF : Outport  Port=5
  wires:
  Rate Transition3/1 -> Product1/2
  Rate Transition2/1 -> Fourier1/1, Fourier/1, Product1/1
  Vac/1 -> Rate Transition/1
  Rate Transition/1 -> Product/1, Power/1
  Idc/1 -> Rate Transition3/1
  Vdc/1 -> Rate Transition2/1
  Rate Transition1/1 -> Product/2, THD2/1, Power/2
  Divide2/1 -> PF/1
  Sqrt/1 -> Divide2/2
  Add/1 -> Sqrt/1
  Math Function2/1 -> Add/2
  Math Function1/1 -> Add/1
  Power/2 -> Math Function2/1
  Power/1 -> Divide2/1, Math Function1/1
  Gain3/1 -> Ripple%/1, Scope3/4  "Vdc Ripple (%)"
  Fourier1/2 -> Terminator/1
  Gain4/1 -> Divide/1
  Fourier1/1 -> Gain4/1
  Divide/1 -> Gain3/1
  Saturation/1 -> Divide/2, Vdc_mean/1, Scope3/2
  Fourier/1 -> Saturation/1
  Fourier/2 -> Terminator1/1
  Mean2/1 -> THD%/1, Scope3/3  "Iac THD (%)"
  Gain2/1 -> Mean2/1
  Mux2/1 -> Pac_Pdc_kW/1, Scope3/1  "Pac  Pdc"
  Iac/1 -> Rate Transition1/1
  Mean1/1 -> Gain1/1
  THD2/1 -> Gain2/1
  Gain/1 -> Mux2/1  "Pac_kW"
  Product/1 -> Mean/1
  Mean/1 -> Gain/1
  Product1/1 -> Mean1/1
  Gain1/1 -> Mux2/2  "Vdc mean"
